simulink model "vrcrane_joystick"  (Simulink 7.4)
settings: Solver=ode45  StartTime=0.0  StopTime=inf  RelTol=1e-3
PostLoadFcn:
  | Ra=2.6;
  | La=0.012;
  | B=1e-1;
  | Kt=1e2;
  | Kv=3e-2;
  | Kg=1e-3;
  | J=0.1;
  | g=9.80665;
  | m_head=100;
  | Gamma=10;
libraries: vrlib x7, simulink_extras x6
Description:
  | Portal Crane with Joystick Control
  | 
  | The vrcrane_joystick example illustrates how a Simulink(R) model can interact with
  | a virtual world. The portal crane dynamics is modeled in Simulink and visualized
  | in virtual reality. The model uses Joystick Input block to control the setpoint.
  | Joystick 3 axes are used to control the setpoint position, button 1 is used to start the crane.
  | 
  | In order to minimize the number of signals transferred between the Simulink model
  | and the virtual reality world and to keep the model as simple and flexible as possible,
  | only the minimum set of moving objects properties are sent from the model to the
  | VR Sink block. All other values necessary for describing the virtual reality objects
  | movement are computed from this minimum set using VRMLScript written
  | in the associated VRML file.
  | 
  | For details on how the crane model hierarchy and scripting logic is implemented
  | please view the associated commented VRML file portal_crane.wrl in a text editor.
  | 
  | This example requires a standard Joystick with at least 3 independent axes
  | connected to the PC.
  | 
  | Acknowledgements:
  | 
  | The Portal crane VRML model is based on the work done by Mr. Martin Foltin
  | and Mr. Samuel Bartos, Department of Automatic Control Systems,
  | Slovak Technical University, Bratislava, Slovak Republic.
settings Model: Creator=Danek  LastModifiedBy=Houska
settings DataIOCC: SignalLoggingName=logsOut
settings OptimizationCC: InlineInvariantSignals=on  InitFltsAndDblsToZero=on
settings DebuggingCC: CheckExecutionContextPreStartOutputMsg=on  CheckExecutionContextRuntimeOutputMsg=on  SignalResolutionControl=TryResolveAllWithWarning  MultiTaskDSMMsg=warning  MultiTaskCondExecSysMsg=none  StrictBusMsg=None
settings ModelReferenceCC: UpdateModelReferenceTargets=IfOutOfDate
settings SFSimCC: SimGenerateEmlReport=off
settings RTWCC: IncludeERTFirstTime=on
settings GRTTargetCC: TargetFcnLib=ansi_tfl_tmw.mat

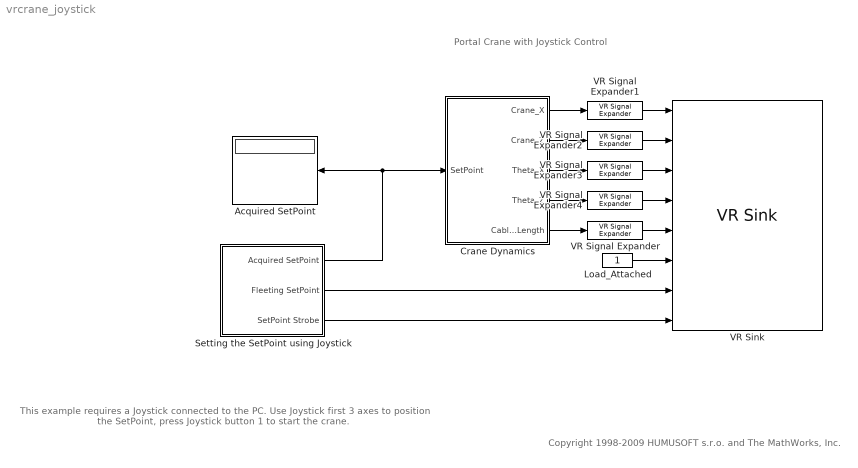
== system vrcrane_joystick ==
  note: Portal Crane with Joystick Control
  note: This example requires a Joystick connected to the PC.
      | Use Joystick first 3 axes to position the SetPoint, press Joystick button 1 to start the crane.
  note: Copyright 1998-2009 HUMUSOFT s.r.o. and The MathWorks, Inc.
  Acquired SetPoint : Display
  Crane Dynamics : Subsystem
  Load_Attached : Constant  OutDataType=sfix(16)  OutScaling=2^0
  Setting the SetPoint using Joystick : Subsystem
      settings: AttributesFormatString=(Joystick ID and Axes\nmust be set properly!)
  VR Signal Expander : vrlib/VR Signal Expander  SystemSampleTime=-1  outwidth=3  outidx=[2]
  VR Signal Expander1 : vrlib/VR Signal Expander  SystemSampleTime=-1  outwidth=3  outidx=[1]
  VR Signal Expander2 : vrlib/VR Signal Expander  SystemSampleTime=-1  outwidth=3  outidx=[3]
  VR Signal Expander3 : vrlib/VR Signal Expander  SystemSampleTime=-1  outwidth=4  outidx=[4]
  VR Signal Expander4 : vrlib/VR Signal Expander  SystemSampleTime=-1  outwidth=4  outidx=[4]
  VR Sink : vrlib/VR Sink  InstantiateOnLoad=on  SampleTime=0.1  ViewEnable=on  RemoteChange=off  RemoteView=off  FieldsWritten=Crane_X.translation.3.1.double#Crane_Z.translation.3.1.double#Parts_Rot_ZAxis.rotation.4.1.double#Parts_Rot_XAxis.rotation.4.1.double#CableUnit.scale.3.1.double#Load_Switch.whichChoice.1.1.double#SetPoint.translation.3.1.double#SP_Highlight.whichChoice.1.1.double  WorldFileName=portal_crane.wrl  WorldDescription=VR Portal Crane  AutoView=on  VideoDimensions=[]  FigureProperties="{'Position', 'Name', 'Viewpoint', 'CameraBound', 'CameraDirection', 'CameraPosition', 'CameraUpVector', 'ZoomFactor', 'Antialiasing', 'Headlight', 'Lighting', 'NavPanel', 'StatusBar', 'ToolBar', 'Textures', 'Transparency', 'Wireframe', 'NavZones', 'NavMode', 'NavSpeed', 'Record2DCompressMethod', 'Record2DCompressQuality', 'Record2D', 'Record2DFileName', 'Record2DFPS'; [1.4000000000000000e+001  7.9000000000000000e+001  5.7600000000000000e+002  3.8000000000000000e+002], 'VR Portal Crane', 'Overview', 'on', [0.0000000000000000e+000  3.1410752802896701e-002 -9.9950656056293852e-001], [-1.7763568394002505e-015 -1.6810838359289786e+000  2.2493946501901263e-001], [0.0000000000000000e+000  9.9950656056293863e-001  3.1410752802896701e-002], [1.0000000000000000e+000], 'off', 'on', 'on', 'halfbar', 'off', 'on', 'on', 'on', 'off', 'off', 'examine', 'normal', 'auto', [7.5000000000000000e+001], 'off', '%f_anim_%n.avi', [1.5000000000000000e+001]}"
  wires:
  Setting the SetPoint using Joystick/1(Acquired SetPoint) -> Acquired SetPoint/1, Crane Dynamics/1(SetPoint)
  Setting the SetPoint using Joystick/2(Fleeting SetPoint) -> VR Sink/7
  Setting the SetPoint using Joystick/3(SetPoint Strobe) -> VR Sink/8
  Load_Attached/1 -> VR Sink/6
  VR Signal Expander/1 -> VR Sink/5
  VR Signal Expander1/1 -> VR Sink/1
  VR Signal Expander2/1 -> VR Sink/2
  VR Signal Expander3/1 -> VR Sink/3
  VR Signal Expander4/1 -> VR Sink/4
  Crane Dynamics/5(Cable_Length) -> VR Signal Expander/1
  Crane Dynamics/1(Crane_X) -> VR Signal Expander1/1
  Crane Dynamics/3(Theta_X) -> VR Signal Expander3/1
  Crane Dynamics/2(Crane_Z) -> VR Signal Expander2/1
  Crane Dynamics/4(Theta_Z) -> VR Signal Expander4/1

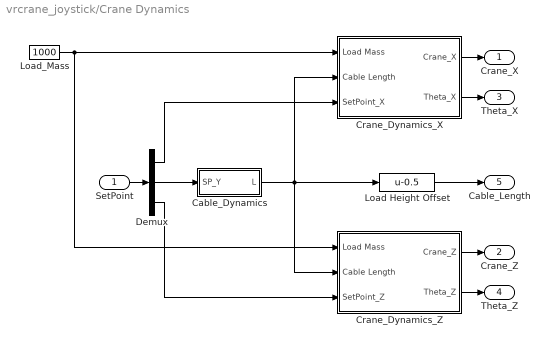
== system vrcrane_joystick/Crane Dynamics ==
  SetPoint : Inport  OutDataType=sfix(16)  OutScaling=2^0
  Cable_Dynamics : Subsystem
  Crane_Dynamics_X : Subsystem
  Crane_Dynamics_Z : Subsystem
  Demux : Demux  Outputs=3
  "Load Height Offset " : Fcn  Expr=u-0.5
  Load_Mass : Constant  Value=1000  OutDataType=sfix(16)  OutScaling=2^0
  Crane_X : Outport  OutDataType=sfix(16)  OutScaling=2^0
  Crane_Z : Outport  Port=2  OutDataType=sfix(16)  OutScaling=2^0
  Theta_X : Outport  Port=3  OutDataType=sfix(16)  OutScaling=2^0
  Theta_Z : Outport  Port=4  OutDataType=sfix(16)  OutScaling=2^0
  Cable_Length : Outport  Port=5  OutDataType=sfix(16)  OutScaling=2^0
  wires:
  Cable_Dynamics/1(L) -> Crane_Dynamics_X/2(Cable Length), Crane_Dynamics_Z/2(Cable Length), "Load Height Offset "/1
  Demux/2 -> Cable_Dynamics/1(SP_Y)
  Demux/1 -> Crane_Dynamics_X/3(SetPoint_X)
  Load_Mass/1 -> Crane_Dynamics_Z/1(Load Mass), Crane_Dynamics_X/1(Load Mass)
  SetPoint/1 -> Demux/1
  Crane_Dynamics_X/1(Crane_X) -> Crane_X/1
  Crane_Dynamics_X/2(Theta_X) -> Theta_X/1
  "Load Height Offset "/1 -> Cable_Length/1
  Crane_Dynamics_Z/1(Crane_Z) -> Crane_Z/1
  Crane_Dynamics_Z/2(Theta_Z) -> Theta_Z/1
  Demux/3 -> Crane_Dynamics_Z/3(SetPoint_Z)

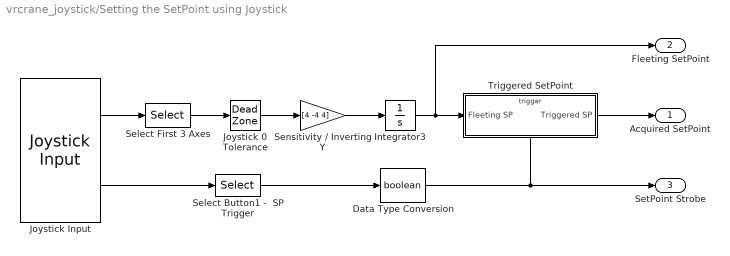
== system vrcrane_joystick/Setting the SetPoint using Joystick ==
  Data Type Conversion : DataTypeConversion  OutDataTypeMode=boolean  OutDataType=sfix(16)  OutScaling=2^0  OutDataTypeStr=boolean
  Integrator3 : Integrator  InitialCondition=[0 0 0]  LimitOutput=on  UpperSaturationLimit=[20 10 20]  LowerSaturationLimit=[0 0 0]
  Joystick 0 Tolerance : DeadZone  LowerValue=-0.3  UpperValue=0.3  SaturateOnIntegerOverflow=on
  Joystick Input : vrlib/Joystick Input  joyid=1  adjustports=off  forcefeed=off
      settings: AttributesFormatString=(Joystick ID and Axes\nmust be set properly!)
  Select Button1 -  SP Trigger : Selector  InputPortWidth=32  IndexOptions=Index vector (dialog)  Indices=[1]  OutputSizes=1
  Select First 3 Axes : Selector  InputPortWidth=8  IndexOptions=Index vector (dialog)  Indices=[1 3 2]  OutputSizes=1
      settings: AttributesFormatString=(Joystick - dependent)
  "Sensitivity / Inverting Y " : Gain  Gain=[4 -4 4]  ParameterDataType=sfix(16)  ParameterScaling=2^0  OutDataType=sfix(16)  OutScaling=2^0
      settings: AttributesFormatString=(Joystick - dependent)
  Triggered SetPoint : Subsystem  TreatAsAtomicUnit=on
  Acquired SetPoint : Outport  OutDataType=sfix(16)  OutScaling=2^0
  Fleeting SetPoint : Outport  Port=2  OutDataType=sfix(16)  OutScaling=2^0
  SetPoint Strobe : Outport  Port=3  OutDataType=sfix(16)  OutScaling=2^0
  wires:
  Triggered SetPoint/1(Triggered SP) -> Acquired SetPoint/1
  Joystick Input/1 -> Select First 3 Axes/1
  Select First 3 Axes/1 -> Joystick 0 Tolerance/1
  Joystick 0 Tolerance/1 -> "Sensitivity / Inverting Y "/1
  Joystick Input/2 -> Select Button1 -  SP Trigger/1
  Integrator3/1 -> Fleeting SetPoint/1, Triggered SetPoint/1(Fleeting SP)
  Select Button1 -  SP Trigger/1 -> Data Type Conversion/1
  "Sensitivity / Inverting Y "/1 -> Integrator3/1
  Data Type Conversion/1 -> SetPoint Strobe/1, Triggered SetPoint/Trigger

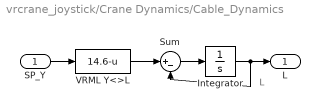
== system vrcrane_joystick/Crane Dynamics/Cable_Dynamics ==
  note: L
  SP_Y : Inport  OutDataType=sfix(16)  OutScaling=2^0
  Integrator : Integrator  InitialCondition=14.6  LimitOutput=on  UpperSaturationLimit=14.6  LowerSaturationLimit=4.6
  Sum : Sum  Inputs=|+-  OutDataType=sfix(16)  OutScaling=2^0
  VRML Y<>L : Fcn  Expr=14.6-u  SampleTime=0
  L : Outport  OutDataType=sfix(16)  OutScaling=2^0
  wires:
  Sum/1 -> Integrator/1
  VRML Y<>L/1 -> Sum/1
  Integrator/1 -> Sum/2, L/1
  SP_Y/1 -> VRML Y<>L/1

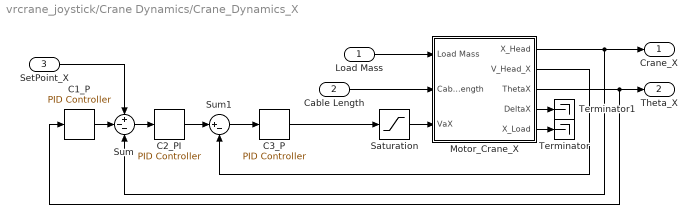
== system vrcrane_joystick/Crane Dynamics/Crane_Dynamics_X ==
  Load Mass : Inport  OutDataType=sfix(16)  OutScaling=2^0
  Cable Length : Inport  Port=2  OutDataType=sfix(16)  OutScaling=2^0
  SetPoint_X : Inport  Port=3  OutDataType=sfix(16)  OutScaling=2^0
  C1_P : simulink_extras/Additional Linear/PID Controller  P=-20  I=0  D=0
  C2_PI : simulink_extras/Additional Linear/PID Controller  P=2.5  I=0  D=0
  C3_P : simulink_extras/Additional Linear/PID Controller  P=5  I=0  D=0
  Motor_Crane_X : Subsystem
  Saturation : Saturate  UpperLimit=50  LowerLimit=-50  OutDataType=sfix(16)  OutScaling=2^0
  Sum : Sum  Inputs=+--  OutDataType=sfix(16)  OutScaling=2^0  SaturateOnIntegerOverflow=on  InputSameDT=on  OutDataTypeStr=Inherit: Same as first input
  Sum1 : Sum  Inputs=|+-  OutDataType=sfix(16)  OutScaling=2^0  SaturateOnIntegerOverflow=on  InputSameDT=on  OutDataTypeStr=Inherit: Same as first input
  Terminator : Terminator
  Terminator1 : Terminator
  Crane_X : Outport  OutDataType=sfix(16)  OutScaling=2^0
  Theta_X : Outport  Port=2  OutDataType=sfix(16)  OutScaling=2^0
  wires:
  Motor_Crane_X/1(X_Head) -> Crane_X/1, Sum/3
  Load Mass/1 -> Motor_Crane_X/1(Load Mass)
  Motor_Crane_X/2(V_Head_X) -> Sum1/2
  Cable Length/1 -> Motor_Crane_X/2(Cable Length)
  Motor_Crane_X/3(ThetaX) -> Theta_X/1, C1_P/1
  Motor_Crane_X/4(DeltaX) -> Terminator1/1
  Motor_Crane_X/5(X_Load) -> Terminator/1
  SetPoint_X/1 -> Sum/1
  Sum/1 -> C2_PI/1
  C2_PI/1 -> Sum1/1
  Sum1/1 -> C3_P/1
  Saturation/1 -> Motor_Crane_X/3(VaX)
  C3_P/1 -> Saturation/1
  C1_P/1 -> Sum/2

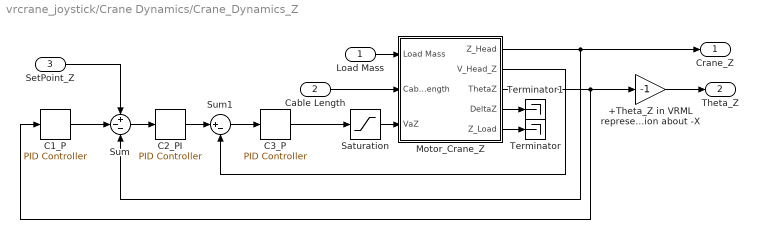
== system vrcrane_joystick/Crane Dynamics/Crane_Dynamics_Z ==
  Load Mass : Inport  OutDataType=sfix(16)  OutScaling=2^0
  Cable Length : Inport  Port=2  OutDataType=sfix(16)  OutScaling=2^0
  SetPoint_Z : Inport  Port=3  OutDataType=sfix(16)  OutScaling=2^0
  +Theta_Z in VRML represented by rotation about -X : Gain  Gain=-1  ParameterDataType=sfix(16)  ParameterScaling=2^0  OutDataType=sfix(16)  OutScaling=2^0
  C1_P : simulink_extras/Additional Linear/PID Controller  P=-20  I=0  D=0
  C2_PI : simulink_extras/Additional Linear/PID Controller  P=2.5  I=0  D=0
  C3_P : simulink_extras/Additional Linear/PID Controller  P=5  I=0  D=0
  Motor_Crane_Z : Subsystem
  Saturation : Saturate  UpperLimit=50  LowerLimit=-50  OutDataType=sfix(16)  OutScaling=2^0
  Sum : Sum  Inputs=+--  OutDataType=sfix(16)  OutScaling=2^0  SaturateOnIntegerOverflow=on  InputSameDT=on  OutDataTypeStr=Inherit: Same as first input
  Sum1 : Sum  Inputs=|+-  OutDataType=sfix(16)  OutScaling=2^0  SaturateOnIntegerOverflow=on  InputSameDT=on  OutDataTypeStr=Inherit: Same as first input
  Terminator : Terminator
  Terminator1 : Terminator
  Crane_Z : Outport  OutDataType=sfix(16)  OutScaling=2^0
  Theta_Z : Outport  Port=2  OutDataType=sfix(16)  OutScaling=2^0
  wires:
  Motor_Crane_Z/1(Z_Head) -> Crane_Z/1, Sum/3
  Load Mass/1 -> Motor_Crane_Z/1(Load Mass)
  Cable Length/1 -> Motor_Crane_Z/2(Cable Length)
  Motor_Crane_Z/3(ThetaZ) -> +Theta_Z in VRML represented by rotation about -X/1, C1_P/1
  Motor_Crane_Z/4(DeltaZ) -> Terminator1/1
  Motor_Crane_Z/5(Z_Load) -> Terminator/1
  Saturation/1 -> Motor_Crane_Z/3(VaZ)
  C3_P/1 -> Saturation/1
  +Theta_Z in VRML represented by rotation about -X/1 -> Theta_Z/1
  Motor_Crane_Z/2(V_Head_Z) -> Sum1/2
  Sum/1 -> C2_PI/1
  C2_PI/1 -> Sum1/1
  Sum1/1 -> C3_P/1
  C1_P/1 -> Sum/2
  SetPoint_Z/1 -> Sum/1

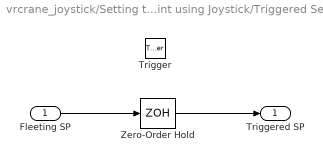
== system vrcrane_joystick/Setting the SetPoint using Joystick/Triggered SetPoint ==
  Fleeting SP : Inport  OutDataType=sfix(16)  OutScaling=2^0
  Trigger : TriggerPort
  Zero-Order Hold : ZeroOrderHold  SampleTime=-1
  Triggered SP : Outport  OutDataType=sfix(16)  OutScaling=2^0
  wires:
  Zero-Order Hold/1 -> Triggered SP/1
  Fleeting SP/1 -> Zero-Order Hold/1

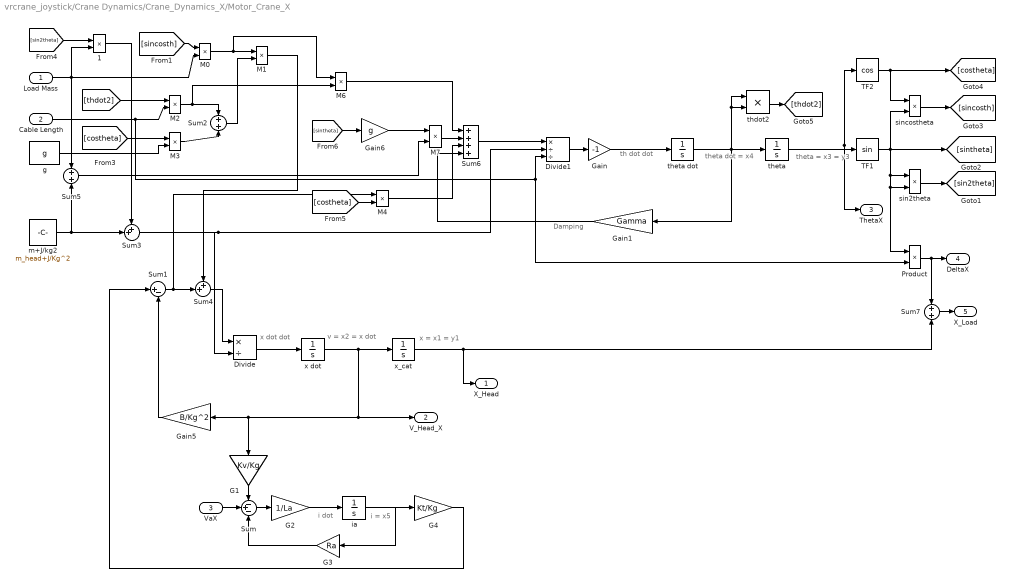
== system vrcrane_joystick/Crane Dynamics/Crane_Dynamics_X/Motor_Crane_X ==
  note: i dot
  note: i = x5
  note: x = x1 = y1
  note: v = x2 = x dot
  note: theta = x3 = y3
  note: theta dot = x4
  note: x dot dot
  note: th dot dot
  note: Damping
  Load Mass : Inport  OutDataType=sfix(16)  OutScaling=2^0
  Cable Length : Inport  Port=2  OutDataType=sfix(16)  OutScaling=2^0
  VaX : Inport  Port=3  OutDataType=sfix(16)  OutScaling=2^0
  " 1" : Product  Inputs=**  OutDataType=sfix(16)  OutScaling=2^-10
  Divide : Product  Inputs=*/  OutDataType=sfix(16)  OutScaling=2^-10
  Divide1 : Product  Inputs=*//  OutDataType=sfix(16)  OutScaling=2^-10
  G1 : Gain  Gain=Kv/Kg  ParameterDataType=sfix(16)  ParameterScaling=2^0  OutDataType=sfix(16)  OutScaling=2^0
  G2 : Gain  Gain=1/La  ParameterDataType=sfix(16)  ParameterScaling=2^0  OutDataType=sfix(16)  OutScaling=2^0
  G3 : Gain  Gain=Ra  ParameterDataType=sfix(16)  ParameterScaling=2^0  OutDataType=sfix(16)  OutScaling=2^0
  G4 : Gain  Gain=Kt/Kg  ParameterDataType=sfix(16)  ParameterScaling=2^0  OutDataType=sfix(16)  OutScaling=2^0
  Gain : Gain  Gain=-1  ParameterDataType=sfix(16)  ParameterScaling=2^0  OutDataType=sfix(16)  OutScaling=2^0
  Gain1 : Gain  Gain=Gamma  ParameterDataType=sfix(16)  ParameterScaling=2^0  OutDataType=sfix(16)  OutScaling=2^0
  Gain5 : Gain  Gain=B/Kg^2  ParameterDataType=sfix(16)  ParameterScaling=2^0  OutDataType=sfix(16)  OutScaling=2^0
  Gain6 : Gain  Gain=g  ParameterDataType=sfix(16)  ParameterScaling=2^0  OutDataType=sfix(16)  OutScaling=2^0
  M{0..4,6..7} (7 alike) : Product  Inputs=**  OutDataType=sfix(16)  OutScaling=2^-10
  Product : Product  OutDataType=sfix(16)  OutScaling=2^0  SaturateOnIntegerOverflow=on  OutDataTypeStr=Inherit: Same as first input
  Sum : Sum  Inputs=-+-  OutDataType=sfix(16)  OutScaling=2^0
  Sum1 : Sum  Inputs=|+-  OutDataType=sfix(16)  OutScaling=2^0
  Sum2 : Sum  OutDataType=sfix(16)  OutScaling=2^0
  Sum3 : Sum  Inputs=++|  OutDataType=sfix(16)  OutScaling=2^0
  Sum4 : Sum  Inputs=++|  OutDataType=sfix(16)  OutScaling=2^0
  Sum5 : Sum  OutDataType=sfix(16)  OutScaling=2^0
  Sum6 : Sum  Inputs=++++  OutDataType=sfix(16)  OutScaling=2^0
  Sum7 : Sum  OutDataType=sfix(16)  OutScaling=2^0
  TF1 : Trigonometry
  TF2 : Trigonometry  Operator=cos
  g : Constant  Value=g  OutDataType=sfix(16)  OutScaling=2^0
  ia : Integrator
  m+J/kg2 : Constant  Value=m_head+J/Kg^2  OutDataType=sfix(16)  OutScaling=2^0
  sin2theta : Product  Inputs=**  OutDataType=sfix(16)  OutScaling=2^-10
  sincostheta : Product  Inputs=**  OutDataType=sfix(16)  OutScaling=2^-10
  thdot2 : Product  Inputs=**  OutDataType=sfix(16)  OutScaling=2^-10
  theta : Integrator
  theta dot : Integrator
  x dot : Integrator
  x_cat : Integrator
  X_Head : Outport  OutDataType=sfix(16)  OutScaling=2^0
  V_Head_X : Outport  Port=2  OutDataType=sfix(16)  OutScaling=2^0
  ThetaX : Outport  Port=3  OutDataType=sfix(16)  OutScaling=2^0
  DeltaX : Outport  Port=4  OutDataType=sfix(16)  OutScaling=2^0
  X_Load : Outport  Port=5  OutDataType=sfix(16)  OutScaling=2^0
  wires:
  G1/1 -> Sum/1
  Sum/1 -> G2/1
  G2/1 -> ia/1
  ia/1 -> G3/1, G4/1
  G3/1 -> Sum/3
  x dot/1 -> x_cat/1, G1/1, Gain5/1, V_Head_X/1
  theta/1 -> ThetaX/1, TF1/1, TF2/1
  theta dot/1 -> theta/1, thdot2/2, thdot2/1, Gain1/1
  G4/1 -> Sum1/1
  Divide/1 -> x dot/1
  Gain5/1 -> Sum1/2
  sin2theta/1 -> [sin2theta]
  sincostheta/1 -> [sincosth]
  [sincosth] -> M0/1
  Load Mass/1 -> Sum5/1, M0/2, " 1"/2
  thdot2/1 -> [thdot2]
  M0/1 -> M1/1, M6/1
  [thdot2] -> M2/1
  [costheta] -> M3/1
  g/1 -> M3/2
  M3/1 -> Sum2/2
  Sum2/1 -> M1/2
  [sin2theta] -> " 1"/1
  " 1"/1 -> Sum3/1
  Sum3/1 -> Divide1/2, Divide/2
  Sum4/1 -> Divide/1
  M1/1 -> Sum4/1
  Sum1/1 -> Sum4/2, M4/1
  M2/1 -> Sum2/1, M6/2
  M6/1 -> Sum6/1
  [costheta] -> M4/2
  Sum5/1 -> M7/2
  [sintheta] -> Gain6/1
  Gain6/1 -> M7/1
  M7/1 -> Sum6/2
  M4/1 -> Sum6/3
  Sum6/1 -> Divide1/1
  Cable Length/1 -> M2/2, Divide1/3, Product/2
  Divide1/1 -> Gain/1
  Gain/1 -> theta dot/1
  x_cat/1 -> X_Head/1, Sum7/2
  VaX/1 -> Sum/2
  m+J/kg2/1 -> Sum3/2, Sum5/2
  Product/1 -> DeltaX/1, Sum7/1
  TF2/1 -> [costheta], sincostheta/1
  TF1/1 -> [sintheta], sincostheta/2, sin2theta/2, Product/1, sin2theta/1
  Sum7/1 -> X_Load/1
  Gain1/1 -> Sum6/4

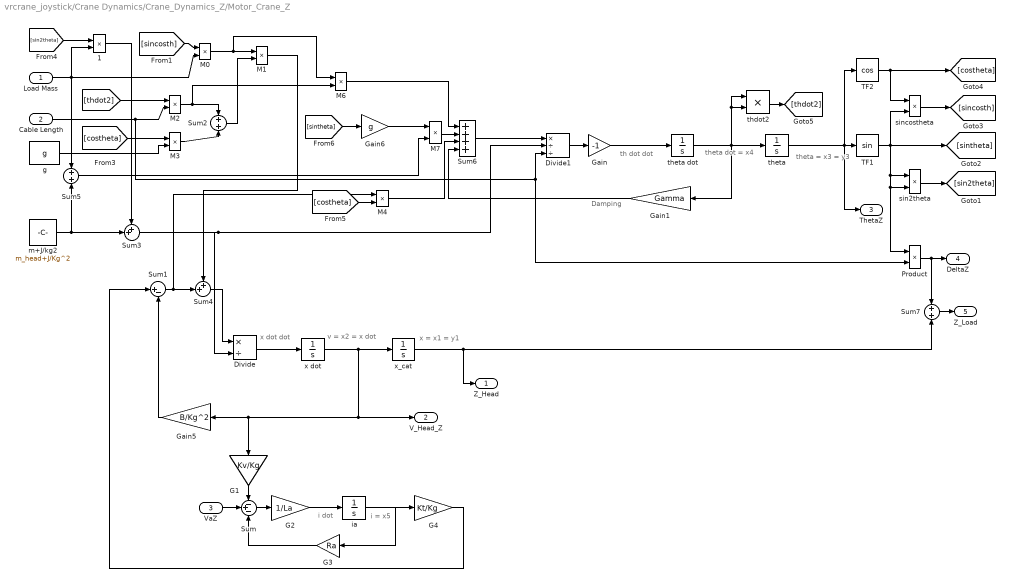
== system vrcrane_joystick/Crane Dynamics/Crane_Dynamics_Z/Motor_Crane_Z ==
  note: i dot
  note: i = x5
  note: x = x1 = y1
  note: v = x2 = x dot
  note: theta = x3 = y3
  note: theta dot = x4
  note: x dot dot
  note: th dot dot
  note: Damping
  Load Mass : Inport  OutDataType=sfix(16)  OutScaling=2^0
  Cable Length : Inport  Port=2  OutDataType=sfix(16)  OutScaling=2^0
  VaZ : Inport  Port=3  OutDataType=sfix(16)  OutScaling=2^0
  " 1" : Product  Inputs=**  OutDataType=sfix(16)  OutScaling=2^-10
  Divide : Product  Inputs=*/  OutDataType=sfix(16)  OutScaling=2^-10
  Divide1 : Product  Inputs=*//  OutDataType=sfix(16)  OutScaling=2^-10
  G1 : Gain  Gain=Kv/Kg  ParameterDataType=sfix(16)  ParameterScaling=2^0  OutDataType=sfix(16)  OutScaling=2^0
  G2 : Gain  Gain=1/La  ParameterDataType=sfix(16)  ParameterScaling=2^0  OutDataType=sfix(16)  OutScaling=2^0
  G3 : Gain  Gain=Ra  ParameterDataType=sfix(16)  ParameterScaling=2^0  OutDataType=sfix(16)  OutScaling=2^0
  G4 : Gain  Gain=Kt/Kg  ParameterDataType=sfix(16)  ParameterScaling=2^0  OutDataType=sfix(16)  OutScaling=2^0
  Gain : Gain  Gain=-1  ParameterDataType=sfix(16)  ParameterScaling=2^0  OutDataType=sfix(16)  OutScaling=2^0
  Gain1 : Gain  Gain=Gamma  ParameterDataType=sfix(16)  ParameterScaling=2^0  OutDataType=sfix(16)  OutScaling=2^0
  Gain5 : Gain  Gain=B/Kg^2  ParameterDataType=sfix(16)  ParameterScaling=2^0  OutDataType=sfix(16)  OutScaling=2^0
  Gain6 : Gain  Gain=g  ParameterDataType=sfix(16)  ParameterScaling=2^0  OutDataType=sfix(16)  OutScaling=2^0
  M{0..4,6..7} (7 alike) : Product  Inputs=**  OutDataType=sfix(16)  OutScaling=2^-10
  Product : Product  OutDataType=sfix(16)  OutScaling=2^0  SaturateOnIntegerOverflow=on  OutDataTypeStr=Inherit: Same as first input
  Sum : Sum  Inputs=-+-  OutDataType=sfix(16)  OutScaling=2^0
  Sum1 : Sum  Inputs=|+-  OutDataType=sfix(16)  OutScaling=2^0
  Sum2 : Sum  OutDataType=sfix(16)  OutScaling=2^0
  Sum3 : Sum  Inputs=++|  OutDataType=sfix(16)  OutScaling=2^0
  Sum4 : Sum  Inputs=++|  OutDataType=sfix(16)  OutScaling=2^0
  Sum5 : Sum  OutDataType=sfix(16)  OutScaling=2^0
  Sum6 : Sum  Inputs=++++  OutDataType=sfix(16)  OutScaling=2^0
  Sum7 : Sum  OutDataType=sfix(16)  OutScaling=2^0
  TF1 : Trigonometry
  TF2 : Trigonometry  Operator=cos
  g : Constant  Value=g  OutDataType=sfix(16)  OutScaling=2^0
  ia : Integrator
  m+J/kg2 : Constant  Value=m_head+J/Kg^2  OutDataType=sfix(16)  OutScaling=2^0
  sin2theta : Product  Inputs=**  OutDataType=sfix(16)  OutScaling=2^-10
  sincostheta : Product  Inputs=**  OutDataType=sfix(16)  OutScaling=2^-10
  thdot2 : Product  Inputs=**  OutDataType=sfix(16)  OutScaling=2^-10
  theta : Integrator
  theta dot : Integrator
  x dot : Integrator
  x_cat : Integrator
  Z_Head : Outport  OutDataType=sfix(16)  OutScaling=2^0
  V_Head_Z : Outport  Port=2  OutDataType=sfix(16)  OutScaling=2^0
  ThetaZ : Outport  Port=3  OutDataType=sfix(16)  OutScaling=2^0
  DeltaZ : Outport  Port=4  OutDataType=sfix(16)  OutScaling=2^0
  Z_Load : Outport  Port=5  OutDataType=sfix(16)  OutScaling=2^0
  wires:
  G1/1 -> Sum/1
  Sum/1 -> G2/1
  G2/1 -> ia/1
  ia/1 -> G3/1, G4/1
  G3/1 -> Sum/3
  x dot/1 -> x_cat/1, G1/1, Gain5/1, V_Head_Z/1
  theta/1 -> ThetaZ/1, TF1/1, TF2/1
  theta dot/1 -> theta/1, thdot2/2, thdot2/1, Gain1/1
  G4/1 -> Sum1/1
  Divide/1 -> x dot/1
  Gain5/1 -> Sum1/2
  sin2theta/1 -> [sin2theta]
  sincostheta/1 -> [sincosth]
  [sincosth] -> M0/1
  Load Mass/1 -> Sum5/1, M0/2, " 1"/2
  thdot2/1 -> [thdot2]
  M0/1 -> M1/1, M6/1
  [thdot2] -> M2/1
  [costheta] -> M3/1
  g/1 -> M3/2
  M3/1 -> Sum2/2
  Sum2/1 -> M1/2
  [sin2theta] -> " 1"/1
  " 1"/1 -> Sum3/1
  Sum3/1 -> Divide1/2, Divide/2
  Sum4/1 -> Divide/1
  M1/1 -> Sum4/1
  Sum1/1 -> Sum4/2, M4/1
  M2/1 -> Sum2/1, M6/2
  M6/1 -> Sum6/1
  [costheta] -> M4/2
  Sum5/1 -> M7/2
  [sintheta] -> Gain6/1
  Gain6/1 -> M7/1
  M7/1 -> Sum6/2
  M4/1 -> Sum6/3
  Sum6/1 -> Divide1/1
  Cable Length/1 -> M2/2, Divide1/3, Product/2
  Divide1/1 -> Gain/1
  Gain/1 -> theta dot/1
  x_cat/1 -> Z_Head/1, Sum7/2
  VaZ/1 -> Sum/2
  m+J/kg2/1 -> Sum3/2, Sum5/2
  Product/1 -> DeltaZ/1, Sum7/1
  TF2/1 -> [costheta], sincostheta/1
  TF1/1 -> [sintheta], sincostheta/2, sin2theta/2, Product/1, sin2theta/1
  Sum7/1 -> Z_Load/1
  Gain1/1 -> Sum6/4
